simulink model "task1c"  (R2015b)
settings: Solver=FixedStepAuto  SolverMode=SingleTasking  StartTime=0.0  StopTime=Tsim  FixedStep=Ts  RelTol=1e-3
values from neighbouring files (symbols this model uses):
  g = 9.8    [lab_task1.m]
  l = l_hat_linf    [lab_task1.m]
  x0 = [x2(1); x3(1)]    [lab_task1.m]
settings Model: Creator=palmisanom  LastModifiedBy=kailintong
settings DataIOCC: LimitDataPoints=off
settings DebuggingCC: AllowSymbolicDim=on  SFUnexpectedBacktrackingDiag=error  SFNoUnconditionalDefaultTransitionDiag=error
settings ModelReferenceCC: PropagateSignalLabelsOutOfModel=on
settings SFSimCC: SimUseLocalCustomCode=on
settings RTWCC: RTWUseLocalCustomCode=on
settings GRTTargetCC: TargetLangStandard=C99 (ISO)
settings ConfigComp: CovMetricSettings=dwe  CovHtmlReporting=off  CovSaveCumulativeToWorkspaceVar=off  CovSaveSingleToWorkspaceVar=off  CovModelRefEnable=Off  CovExternalEMLEnable=on

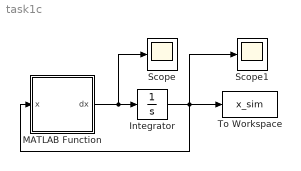
== system task1c ==
  Integrator : Integrator  InitialCondition=x0
  MATLAB Function : MATLAB Function  TreatAsAtomicUnit=on
  Scope : Scope
  Scope1 : Scope
  To Workspace : ToWorkspace  VariableName=x_sim  SaveFormat=Structure With Time  SampleTime=-1
  wires:
  MATLAB Function/1(dx) -> Scope/1, Integrator/1
  Integrator/1 -> MATLAB Function/1(x), Scope1/1, To Workspace/1

== matlab function task1c/MATLAB Function ==
  data: x input; g parameter; dx output; l parameter
function dx = fcn(x,g,l)
dx = [0;0];

dx(1) = x(2);
dx(2) = g/l * (sin(x(1)));
